simulink model "lab2_model_PIDEmulation211_213"  (R2024b)
settings: Solver=FixedStepAuto  StartTime=0.0  StopTime=sIn.simulation_time  FixedStep=1e-4
undefined symbols (not defined in the file or in its folder): degs2rpm, denZOH1, denZOH10, denZOH50, DiscIntNeverNeededParam, drv, filt, gbox, mld, mot, numZOH1, numZOH10, numZOH50, PID, rads2rpm, rpm2degs, sens, sIn, specs
libraries: simulink_extras x24, simulink x4
(part 2 of 2)

== system lab2_model_PIDEmulation211_213/Selfmade model of the Quanser SRV-02 + NI DAQ4/Voltage driver ==
  u[V] : Inport
  Saturation : Saturate  UpperLimit=12  LowerLimit=-12
  Transfer Fcn : TransferFcn  Numerator=[drv.dcgain]  Denominator=[drv.Tc 1]
  udrv[v] : Outport
  wires:
  u[V]/1 -> Transfer Fcn/1
  Transfer Fcn/1 -> Saturation/1
  Saturation/1 -> udrv[v]/1

== system lab2_model_PIDEmulation211_213/Selfmade model of the Quanser SRV-02 + NI DAQ5/DAC ==
  u[V] : Inport
  Quantizer : Quantizer  QuantizationInterval=daq.dac.q
  Saturation : Saturate  UpperLimit=10  LowerLimit=-10
  Zero-Order Hold : ZeroOrderHold  SampleTime=1e-3
  udrv[V] : Outport
  wires:
  Zero-Order Hold/1 -> Quantizer/1
  u[V]/1 -> Zero-Order Hold/1
  Quantizer/1 -> Saturation/1
  Saturation/1 -> udrv[V]/1

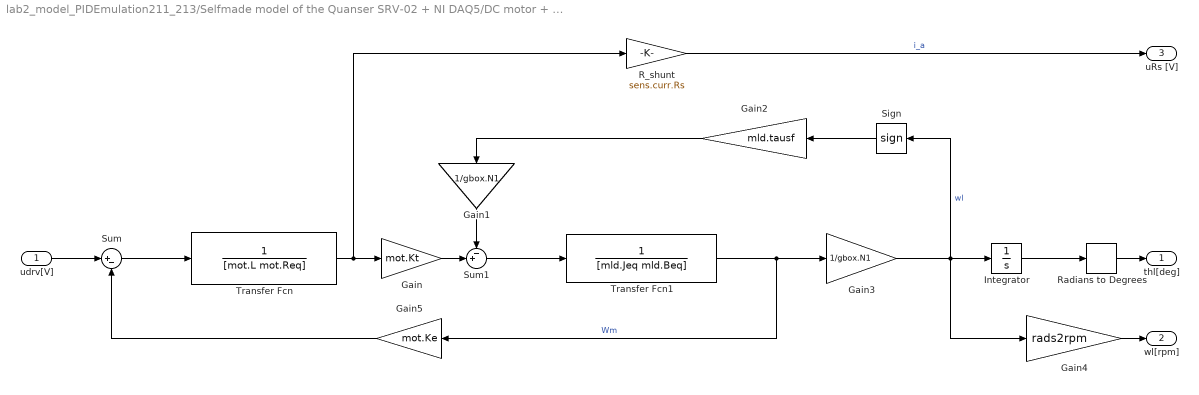
== system lab2_model_PIDEmulation211_213/Selfmade model of the Quanser SRV-02 + NI DAQ5/DC motor + gearbox ==
  udrv[V] : Inport
  Gain : Gain  Gain=mot.Kt
  Gain1 : Gain  Gain=1/gbox.N1
  Gain2 : Gain  Gain=mld.tausf
  Gain3 : Gain  Gain=1/gbox.N1
  Gain4 : Gain  Gain=rads2rpm
  Gain5 : Gain  Gain=mot.Ke
  Integrator : Integrator
  R_shunt : Gain  Gain=sens.curr.Rs
  Radians to Degrees : simulink_extras/Transformations/Radians to Degrees
  Sign : Signum  ZeroCross=off
  Sum : Sum  Inputs=|+-
  Sum1 : Sum  Inputs=-+|
  Transfer Fcn : TransferFcn  Denominator=[mot.L mot.Req]
  Transfer Fcn1 : TransferFcn  Denominator=[mld.Jeq mld.Beq]
  thl[deg] : Outport
  wl[rpm] : Outport  Port=2
  uRs [V] : Outport  Port=3
  wires:
  udrv[V]/1 -> Sum/1
  Sum/1 -> Transfer Fcn/1
  Transfer Fcn/1 -> R_shunt/1, Gain/1
  Gain1/1 -> Sum1/1
  Gain2/1 -> Gain1/1
  Sign/1 -> Gain2/1
  Transfer Fcn1/1 -> Gain5/1, Gain3/1  "Wm"
  Gain3/1 -> Gain4/1, Sign/1, Integrator/1  "wl"
  Integrator/1 -> Radians to Degrees/1
  Radians to Degrees/1 -> thl[deg]/1
  Gain4/1 -> wl[rpm]/1
  Sum1/1 -> Transfer Fcn1/1
  Gain/1 -> Sum1/2
  Gain5/1 -> Sum/2
  R_shunt/1 -> uRs [V]/1  "i_a"

== system lab2_model_PIDEmulation211_213/Selfmade model of the Quanser SRV-02 + NI DAQ5/Encoder ==
  thl[deg] : Inport
  Gain : Gain  Gain=1/sens.enc.pulse2deg
  Quantizer : Quantizer  QuantizationInterval=sens.enc.pulse2deg
  Zero-Order Hold : ZeroOrderHold  SampleTime=1e-3
  thl[pulses] : Outport
  wires:
  thl[deg]/1 -> Zero-Order Hold/1
  Gain/1 -> thl[pulses]/1
  Quantizer/1 -> Gain/1
  Zero-Order Hold/1 -> Quantizer/1

== system lab2_model_PIDEmulation211_213/Selfmade model of the Quanser SRV-02 + NI DAQ5/Voltage driver ==
  u[V] : Inport
  Saturation : Saturate  UpperLimit=12  LowerLimit=-12
  Transfer Fcn : TransferFcn  Numerator=[drv.dcgain]  Denominator=[drv.Tc 1]
  udrv[v] : Outport
  wires:
  u[V]/1 -> Transfer Fcn/1
  Transfer Fcn/1 -> Saturation/1
  Saturation/1 -> udrv[v]/1

== system lab2_model_PIDEmulation211_213/Selfmade model of the Quanser SRV-02 + NI DAQ6/DAC ==
  u[V] : Inport
  Quantizer : Quantizer  QuantizationInterval=daq.dac.q
  Saturation : Saturate  UpperLimit=10  LowerLimit=-10
  Zero-Order Hold : ZeroOrderHold  SampleTime=1e-3
  udrv[V] : Outport
  wires:
  Zero-Order Hold/1 -> Quantizer/1
  u[V]/1 -> Zero-Order Hold/1
  Quantizer/1 -> Saturation/1
  Saturation/1 -> udrv[V]/1

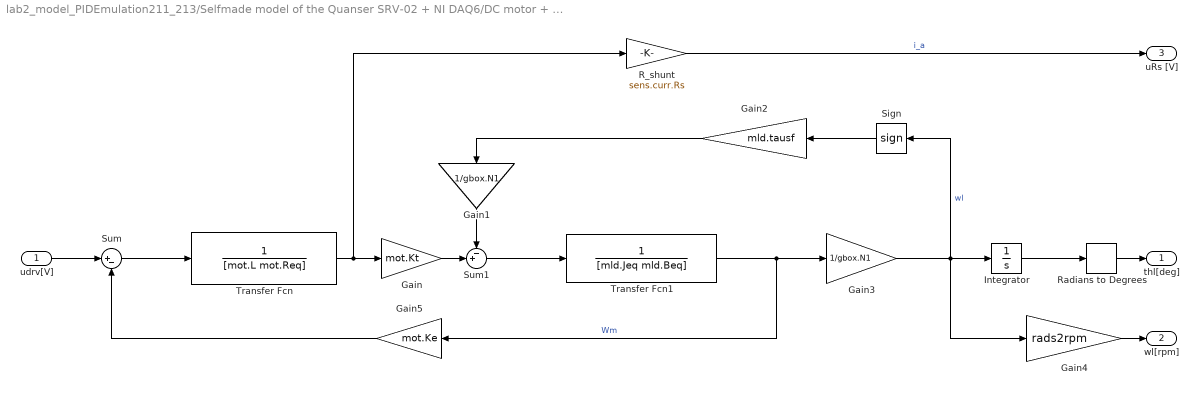
== system lab2_model_PIDEmulation211_213/Selfmade model of the Quanser SRV-02 + NI DAQ6/DC motor + gearbox ==
  udrv[V] : Inport
  Gain : Gain  Gain=mot.Kt
  Gain1 : Gain  Gain=1/gbox.N1
  Gain2 : Gain  Gain=mld.tausf
  Gain3 : Gain  Gain=1/gbox.N1
  Gain4 : Gain  Gain=rads2rpm
  Gain5 : Gain  Gain=mot.Ke
  Integrator : Integrator
  R_shunt : Gain  Gain=sens.curr.Rs
  Radians to Degrees : simulink_extras/Transformations/Radians to Degrees
  Sign : Signum  ZeroCross=off
  Sum : Sum  Inputs=|+-
  Sum1 : Sum  Inputs=-+|
  Transfer Fcn : TransferFcn  Denominator=[mot.L mot.Req]
  Transfer Fcn1 : TransferFcn  Denominator=[mld.Jeq mld.Beq]
  thl[deg] : Outport
  wl[rpm] : Outport  Port=2
  uRs [V] : Outport  Port=3
  wires:
  udrv[V]/1 -> Sum/1
  Sum/1 -> Transfer Fcn/1
  Transfer Fcn/1 -> R_shunt/1, Gain/1
  Gain1/1 -> Sum1/1
  Gain2/1 -> Gain1/1
  Sign/1 -> Gain2/1
  Transfer Fcn1/1 -> Gain5/1, Gain3/1  "Wm"
  Gain3/1 -> Gain4/1, Sign/1, Integrator/1  "wl"
  Integrator/1 -> Radians to Degrees/1
  Radians to Degrees/1 -> thl[deg]/1
  Gain4/1 -> wl[rpm]/1
  Sum1/1 -> Transfer Fcn1/1
  Gain/1 -> Sum1/2
  Gain5/1 -> Sum/2
  R_shunt/1 -> uRs [V]/1  "i_a"

== system lab2_model_PIDEmulation211_213/Selfmade model of the Quanser SRV-02 + NI DAQ6/Encoder ==
  thl[deg] : Inport
  Gain : Gain  Gain=1/sens.enc.pulse2deg
  Quantizer : Quantizer  QuantizationInterval=sens.enc.pulse2deg
  Zero-Order Hold : ZeroOrderHold  SampleTime=1e-3
  thl[pulses] : Outport
  wires:
  thl[deg]/1 -> Zero-Order Hold/1
  Gain/1 -> thl[pulses]/1
  Quantizer/1 -> Gain/1
  Zero-Order Hold/1 -> Quantizer/1

== system lab2_model_PIDEmulation211_213/Selfmade model of the Quanser SRV-02 + NI DAQ6/Voltage driver ==
  u[V] : Inport
  Saturation : Saturate  UpperLimit=12  LowerLimit=-12
  Transfer Fcn : TransferFcn  Numerator=[drv.dcgain]  Denominator=[drv.Tc 1]
  udrv[v] : Outport
  wires:
  u[V]/1 -> Transfer Fcn/1
  Transfer Fcn/1 -> Saturation/1
  Saturation/1 -> udrv[v]/1

== system lab2_model_PIDEmulation211_213/Selfmade model of the Quanser SRV-02 + NI DAQ7/DAC ==
  u[V] : Inport
  Quantizer : Quantizer  QuantizationInterval=daq.dac.q
  Saturation : Saturate  UpperLimit=10  LowerLimit=-10
  Zero-Order Hold : ZeroOrderHold  SampleTime=1e-3
  udrv[V] : Outport
  wires:
  Zero-Order Hold/1 -> Quantizer/1
  u[V]/1 -> Zero-Order Hold/1
  Quantizer/1 -> Saturation/1
  Saturation/1 -> udrv[V]/1

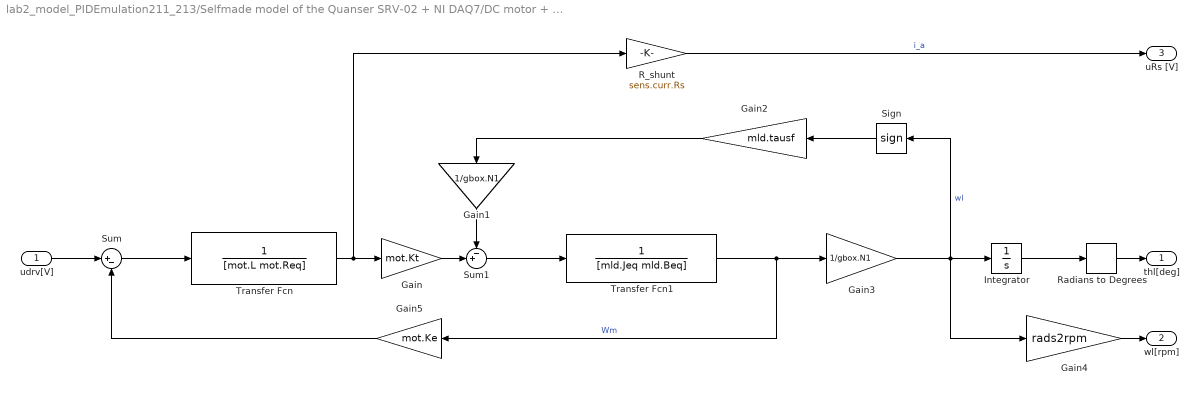
== system lab2_model_PIDEmulation211_213/Selfmade model of the Quanser SRV-02 + NI DAQ7/DC motor + gearbox ==
  udrv[V] : Inport
  Gain : Gain  Gain=mot.Kt
  Gain1 : Gain  Gain=1/gbox.N1
  Gain2 : Gain  Gain=mld.tausf
  Gain3 : Gain  Gain=1/gbox.N1
  Gain4 : Gain  Gain=rads2rpm
  Gain5 : Gain  Gain=mot.Ke
  Integrator : Integrator
  R_shunt : Gain  Gain=sens.curr.Rs
  Radians to Degrees : simulink_extras/Transformations/Radians to Degrees
  Sign : Signum  ZeroCross=off
  Sum : Sum  Inputs=|+-
  Sum1 : Sum  Inputs=-+|
  Transfer Fcn : TransferFcn  Denominator=[mot.L mot.Req]
  Transfer Fcn1 : TransferFcn  Denominator=[mld.Jeq mld.Beq]
  thl[deg] : Outport
  wl[rpm] : Outport  Port=2
  uRs [V] : Outport  Port=3
  wires:
  udrv[V]/1 -> Sum/1
  Sum/1 -> Transfer Fcn/1
  Transfer Fcn/1 -> R_shunt/1, Gain/1
  Gain1/1 -> Sum1/1
  Gain2/1 -> Gain1/1
  Sign/1 -> Gain2/1
  Transfer Fcn1/1 -> Gain5/1, Gain3/1  "Wm"
  Gain3/1 -> Gain4/1, Sign/1, Integrator/1  "wl"
  Integrator/1 -> Radians to Degrees/1
  Radians to Degrees/1 -> thl[deg]/1
  Gain4/1 -> wl[rpm]/1
  Sum1/1 -> Transfer Fcn1/1
  Gain/1 -> Sum1/2
  Gain5/1 -> Sum/2
  R_shunt/1 -> uRs [V]/1  "i_a"

== system lab2_model_PIDEmulation211_213/Selfmade model of the Quanser SRV-02 + NI DAQ7/Encoder ==
  thl[deg] : Inport
  Gain : Gain  Gain=1/sens.enc.pulse2deg
  Quantizer : Quantizer  QuantizationInterval=sens.enc.pulse2deg
  Zero-Order Hold : ZeroOrderHold  SampleTime=1e-3
  thl[pulses] : Outport
  wires:
  thl[deg]/1 -> Zero-Order Hold/1
  Gain/1 -> thl[pulses]/1
  Quantizer/1 -> Gain/1
  Zero-Order Hold/1 -> Quantizer/1

== system lab2_model_PIDEmulation211_213/Selfmade model of the Quanser SRV-02 + NI DAQ7/Voltage driver ==
  u[V] : Inport
  Saturation : Saturate  UpperLimit=12  LowerLimit=-12
  Transfer Fcn : TransferFcn  Numerator=[drv.dcgain]  Denominator=[drv.Tc 1]
  udrv[v] : Outport
  wires:
  u[V]/1 -> Transfer Fcn/1
  Transfer Fcn/1 -> Saturation/1
  Saturation/1 -> udrv[v]/1

== system lab2_model_PIDEmulation211_213/Selfmade model of the Quanser SRV-02 + NI DAQ8/DAC ==
  u[V] : Inport
  Quantizer : Quantizer  QuantizationInterval=daq.dac.q
  Saturation : Saturate  UpperLimit=10  LowerLimit=-10
  Zero-Order Hold : ZeroOrderHold  SampleTime=1e-3
  udrv[V] : Outport
  wires:
  Zero-Order Hold/1 -> Quantizer/1
  u[V]/1 -> Zero-Order Hold/1
  Quantizer/1 -> Saturation/1
  Saturation/1 -> udrv[V]/1

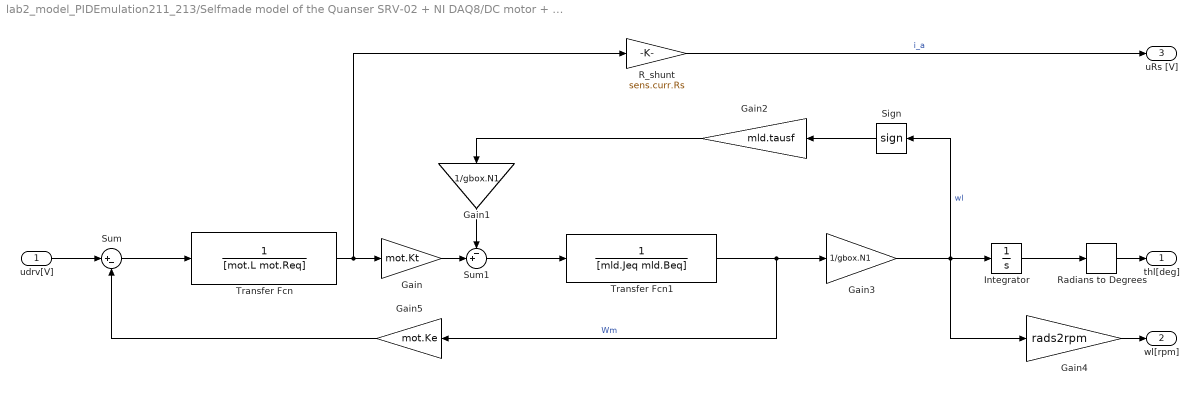
== system lab2_model_PIDEmulation211_213/Selfmade model of the Quanser SRV-02 + NI DAQ8/DC motor + gearbox ==
  udrv[V] : Inport
  Gain : Gain  Gain=mot.Kt
  Gain1 : Gain  Gain=1/gbox.N1
  Gain2 : Gain  Gain=mld.tausf
  Gain3 : Gain  Gain=1/gbox.N1
  Gain4 : Gain  Gain=rads2rpm
  Gain5 : Gain  Gain=mot.Ke
  Integrator : Integrator
  R_shunt : Gain  Gain=sens.curr.Rs
  Radians to Degrees : simulink_extras/Transformations/Radians to Degrees
  Sign : Signum  ZeroCross=off
  Sum : Sum  Inputs=|+-
  Sum1 : Sum  Inputs=-+|
  Transfer Fcn : TransferFcn  Denominator=[mot.L mot.Req]
  Transfer Fcn1 : TransferFcn  Denominator=[mld.Jeq mld.Beq]
  thl[deg] : Outport
  wl[rpm] : Outport  Port=2
  uRs [V] : Outport  Port=3
  wires:
  udrv[V]/1 -> Sum/1
  Sum/1 -> Transfer Fcn/1
  Transfer Fcn/1 -> R_shunt/1, Gain/1
  Gain1/1 -> Sum1/1
  Gain2/1 -> Gain1/1
  Sign/1 -> Gain2/1
  Transfer Fcn1/1 -> Gain5/1, Gain3/1  "Wm"
  Gain3/1 -> Gain4/1, Sign/1, Integrator/1  "wl"
  Integrator/1 -> Radians to Degrees/1
  Radians to Degrees/1 -> thl[deg]/1
  Gain4/1 -> wl[rpm]/1
  Sum1/1 -> Transfer Fcn1/1
  Gain/1 -> Sum1/2
  Gain5/1 -> Sum/2
  R_shunt/1 -> uRs [V]/1  "i_a"

== system lab2_model_PIDEmulation211_213/Selfmade model of the Quanser SRV-02 + NI DAQ8/Encoder ==
  thl[deg] : Inport
  Gain : Gain  Gain=1/sens.enc.pulse2deg
  Quantizer : Quantizer  QuantizationInterval=sens.enc.pulse2deg
  Zero-Order Hold : ZeroOrderHold  SampleTime=1e-3
  thl[pulses] : Outport
  wires:
  thl[deg]/1 -> Zero-Order Hold/1
  Gain/1 -> thl[pulses]/1
  Quantizer/1 -> Gain/1
  Zero-Order Hold/1 -> Quantizer/1

== system lab2_model_PIDEmulation211_213/Selfmade model of the Quanser SRV-02 + NI DAQ8/Voltage driver ==
  u[V] : Inport
  Saturation : Saturate  UpperLimit=12  LowerLimit=-12
  Transfer Fcn : TransferFcn  Numerator=[drv.dcgain]  Denominator=[drv.Tc 1]
  udrv[v] : Outport
  wires:
  u[V]/1 -> Transfer Fcn/1
  Transfer Fcn/1 -> Saturation/1
  Saturation/1 -> udrv[v]/1
